simulink model "AN_Simulink_Model_v1"  (R2019b)
settings: Solver=VariableStepAuto  StartTime=0.0  StopTime=testtime  RelTol=1e-3
InitFcn:
  | AN_InitFcn_Callback
StopFcn:
  | AN_StopFcn_Callback
values from neighbouring files (symbols this model uses):
  C1initphase = C1initphase + atan(CF/(-rzero))-atan((CF-pimag(2*i-1))/(-preal(2*i-1)))-atan((CF+pimag(2*i-1))/(-preal(2*i-1)))    [AN_Get_Model_Parameters.m]
  C1slope = 0.1    [AN_Get_Model_Parameters.m]
  C2slope = 0.2    [AN_Get_Model_Parameters.m]
  CF = 2*pi*cf    [AN_Get_Model_Parameters.m]
  cordiciterationswb = 52    [AN_Get_Model_Parameters.m]
  delta_phase = -2*pi*centerfreq*tdres    [AN_Get_Model_Parameters.m]
  fs_bilinear = 2*pi*cf/tan(2*pi*cf*tdres/2)    [AN_Get_Model_Parameters.m]
  ihcasym = 3.0    (= 3)    [AN_Get_Model_Parameters.m]
  IHCLPcoeffs = [  gainihc*c2LPihc gainihc*c2LPihc 0 1 -c1LPihc 0 ... (first row only)    [AN_Get_Model_Parameters.m]
  MEcoeffs = [m14*m11 m15*m11 m16*m11 1 m12*m11 m13*m11; m24*m21 m25*m21 m26*m21 1 m22*m21 m23*m21; m34*m31 m35*m31 m36*m31 1 m32*m31 m33*m31]    [AN_Get_Model_Parameters.m]
  MEscale = 1/megainmax    (= 0.5)    [AN_Get_Model_Parameters.m]
  minR = minR    (= 0.05)    [AN_Get_Model_Parameters.m]
  norm_gainc1 = single(norm_gainc1)    [AN_Get_Model_Parameters.m]
  OHCLPcoeffs = [gainohc*c2LPohc gainohc*c2LPohc 0 1 -c1LPohc 0; gainohc*c2LPohc gainohc*c2LPohc 0 1 -c1LPohc 0]    [AN_Get_Model_Parameters.m]
  order_of_zero = half_order_pole    (= 5)    [AN_Get_Model_Parameters.m]
  pimag = zeros(11,1)    [AN_Get_Model_Parameters.m]
  preal = zeros(11,1)    [AN_Get_Model_Parameters.m]
  s0 = -dc/log(R1/(1-minR))    [AN_Get_Model_Parameters.m]
  s1 = 5.0    (= 5)    [AN_Get_Model_Parameters.m]
  shift = 1.0/(1.0+ohcasym)    (= 0.125)    [AN_Get_Model_Parameters.m]
  strength = (20.0e6)/(10^(corner/20))    (= 2000)    [AN_Get_Model_Parameters.m]
  tauwb = TauWBMax + (bmTaubm-bmTaumax)*(TauWBMax-TauWBMin)/(bmTaumax-bmTaumin)    [AN_Get_Model_Parameters.m]    (also in AN_StopFcn_Callback.m = TauWBMax+(tauc1(n+1,1)-bmTaumax)*(TauWBMax-TauWBMin)/(bmTaum)
  TauWBMax = Taumin + 0.2*(Taumax-Taumin)    [AN_Get_Model_Parameters.m]
  wborder = 3    [AN_Get_Model_Parameters.m]
  x0 = s0*log((1.0/shift-1)/(1+exp(x1/s1)))    [AN_Get_Model_Parameters.m]
  x1 = 5.0    (= 5)    [AN_Get_Model_Parameters.m]
undefined symbols (not defined in the file or in its folder): bmTaumax, bmTaumin, C2coeffs, cf, cihc, cohc, jsin, norm_gainc2, tdres, wbgain
libraries: simulink x5, dspsrcs4 x1
(part 2 of 2)

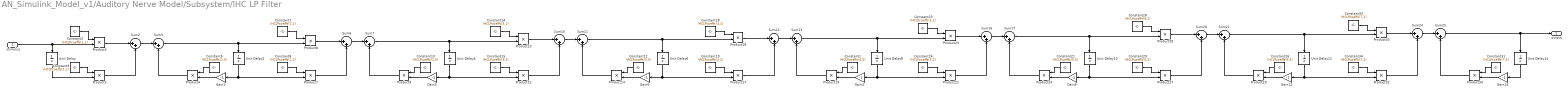
== system AN_Simulink_Model_v1/Auditory Nerve Model/Subsystem/IHC LP Filter ==
  stimulus : Inport  OutDataTypeStr=single
  Constant1 : Constant  Value=IHCLPcoeffs(4,5)  OutDataTypeStr=single  SampleTime=-1
  Constant10 : Constant  Value=IHCLPcoeffs(2,5)  OutDataTypeStr=single  SampleTime=-1
  Constant12 : Constant  Value=IHCLPcoeffs(3,5)  OutDataTypeStr=single  SampleTime=-1
  Constant14 : Constant  Value=IHCLPcoeffs(3,1)  OutDataTypeStr=single  SampleTime=-1
  Constant15 : Constant  Value=IHCLPcoeffs(3,2)  OutDataTypeStr=single  SampleTime=-1
  Constant18 : Constant  Value=IHCLPcoeffs(4,1)  OutDataTypeStr=single  SampleTime=-1
  Constant19 : Constant  Value=IHCLPcoeffs(4,2)  OutDataTypeStr=single  SampleTime=-1
  Constant2 : Constant  Value=IHCLPcoeffs(1,1)  OutDataTypeStr=single  SampleTime=-1
  Constant21 : Constant  Value=IHCLPcoeffs(5,5)  OutDataTypeStr=single  SampleTime=-1
  Constant23 : Constant  Value=IHCLPcoeffs(5,1)  OutDataTypeStr=single  SampleTime=-1
  Constant24 : Constant  Value=IHCLPcoeffs(5,2)  OutDataTypeStr=single  SampleTime=-1
  Constant26 : Constant  Value=IHCLPcoeffs(6,5)  OutDataTypeStr=single  SampleTime=-1
  Constant28 : Constant  Value=IHCLPcoeffs(6,1)  OutDataTypeStr=single  SampleTime=-1
  Constant29 : Constant  Value=IHCLPcoeffs(6,2)  OutDataTypeStr=single  SampleTime=-1
  Constant3 : Constant  Value=IHCLPcoeffs(1,2)  OutDataTypeStr=single  SampleTime=-1
  Constant31 : Constant  Value=IHCLPcoeffs(7,5)  OutDataTypeStr=single  SampleTime=-1
  Constant33 : Constant  Value=IHCLPcoeffs(7,1)  OutDataTypeStr=single  SampleTime=-1
  Constant34 : Constant  Value=IHCLPcoeffs(7,2)  OutDataTypeStr=single  SampleTime=-1
  Constant5 : Constant  Value=IHCLPcoeffs(1,5)  OutDataTypeStr=single  SampleTime=-1
  Constant7 : Constant  Value=IHCLPcoeffs(2,1)  OutDataTypeStr=single  SampleTime=-1
  Constant8 : Constant  Value=IHCLPcoeffs(2,2)  OutDataTypeStr=single  SampleTime=-1
  Gain{1,3..4,6,9,12,14} (7 alike) : Gain  Gain=-1
  Product{2..4,7..9,12..14,17..19,22..24,27..29,32..34} (21 alike) : Product
  Sum{2..3,6..7,10..13,16..17,20..21,24..25} (14 alike) : Sum  Inputs=|++
  Unit Delay{,2,4,6,8,10,12,14} (8 alike) : UnitDelay  SampleTime=-1  HasFrameUpgradeWarning=on
  output : Outport  VectorParamsAs1DForOutWhenUnconnected=off
  wires:
  Unit Delay14/1 -> Gain14/1
  Constant31/1 -> Product34/1
  Product29/1 -> Sum21/2
  Constant33/1 -> Product33/1
  Product13/1 -> Sum10/1
  Product34/1 -> Sum25/2
  Product8/1 -> Sum6/1
  Constant19/1 -> Product17/1
  Gain12/1 -> Product29/2
  Product32/1 -> Sum24/2
  Sum7/1 -> Unit Delay4/1, Product13/2
  Sum21/1 -> Unit Delay12/1, Product33/2
  Sum25/1 -> output/1, Unit Delay14/1
  Gain14/1 -> Product34/2
  Sum24/1 -> Sum25/1
  Product12/1 -> Sum10/2
  Unit Delay2/1 -> Product7/2, Gain1/1
  Unit Delay12/1 -> Product32/2, Gain12/1
  Constant26/1 -> Product29/1
  Product28/1 -> Sum20/1
  Product33/1 -> Sum24/1
  Product19/1 -> Sum13/2
  Product18/1 -> Sum12/1
  Sum16/1 -> Sum17/1
  Product27/1 -> Sum20/2
  Constant34/1 -> Product32/1
  Constant28/1 -> Product28/1
  Unit Delay10/1 -> Product27/2, Gain9/1
  Product24/1 -> Sum17/2
  Unit Delay/1 -> Product2/2
  Sum11/1 -> Unit Delay6/1, Product18/2
  Gain4/1 -> Product19/2
  Constant1/1 -> Product19/1
  stimulus/1 -> Product3/2, Unit Delay/1
  Product4/1 -> Sum3/2
  Constant24/1 -> Product22/1
  Constant21/1 -> Product24/1
  Constant29/1 -> Product27/1
  Gain9/1 -> Product24/2
  Sum20/1 -> Sum21/1
  Sum10/1 -> Sum11/1
  Gain1/1 -> Product4/2
  Unit Delay6/1 -> Product17/2, Gain6/1
  Sum12/1 -> Sum13/1
  Constant15/1 -> Product12/1
  Product14/1 -> Sum11/2
  Unit Delay8/1 -> Product22/2, Gain4/1
  Sum13/1 -> Unit Delay8/1, Product23/2
  Product17/1 -> Sum12/2
  Gain6/1 -> Product14/2
  Constant3/1 -> Product2/1
  Constant8/1 -> Product7/1
  Constant12/1 -> Product14/1
  Product3/1 -> Sum2/1
  Constant14/1 -> Product13/1
  Sum2/1 -> Sum3/1
  Sum17/1 -> Unit Delay10/1, Product28/2
  Product23/1 -> Sum16/1
  Constant10/1 -> Product9/1
  Product9/1 -> Sum7/2
  Constant2/1 -> Product3/1
  Unit Delay4/1 -> Product12/2, Gain3/1
  Product22/1 -> Sum16/2
  Constant18/1 -> Product18/1
  Constant5/1 -> Product4/1
  Constant23/1 -> Product23/1
  Constant7/1 -> Product8/1
  Sum3/1 -> Unit Delay2/1, Product8/2
  Gain3/1 -> Product9/2
  Product2/1 -> Sum2/2
  Sum6/1 -> Sum7/1
  Product7/1 -> Sum6/2

== system AN_Simulink_Model_v1/Auditory Nerve Model/Subsystem1/Calculate tauc1 ==
  note: Calculate final Time Constant which will be fed forward into C1 filter
  In1 : Inport
  Add : Sum
  Constant : Constant  Value=cohc  OutDataTypeStr=single  SampleTime=-1
  Constant1 : Constant  Value=bmTaumin  OutDataTypeStr=single  SampleTime=-1
  Constant2 : Constant  Value=bmTaumin  OutDataTypeStr=single  SampleTime=-1
  Product : Product
  Subtract : Sum  Inputs=+-
  Out1 : Outport  VectorParamsAs1DForOutWhenUnconnected=off
  wires:
  In1/1 -> Subtract/1  "tmptauc1"
  Constant/1 -> Product/1
  Constant1/1 -> Subtract/2
  Product/1 -> Add/1
  Add/1 -> Out1/1  "tauc1"
  Subtract/1 -> Product/2
  Constant2/1 -> Add/2

== system AN_Simulink_Model_v1/Auditory Nerve Model/Subsystem1/NL After OHC Function ==
  note: Ensuring Time Constant Falls within Range
  note: Nonlinear Exponential Function
  stimulus : Inport
  Abs : Abs
  Add3 : Sum
  Constant12 : Constant  Value=minR  OutDataTypeStr=single  SampleTime=-1
  Constant13 : Constant  OutDataTypeStr=single  SampleTime=-1
  Constant14 : Constant  Value=minR  OutDataTypeStr=single  SampleTime=-1
  Constant15 : Constant  Value=bmTaumax  OutDataTypeStr=single  SampleTime=-1
  Constant5 : Constant  Value=s0  OutDataTypeStr=single  SampleTime=-1
  Divide1 : Product  Inputs=*/  SaturateOnIntegerOverflow=on  RndMeth=Zero
  Exp : Math  SaturateOnIntegerOverflow=on
  Gain2 : Gain  Gain=-1
  Product3 : Product
  Product4 : Product
  Saturation : Saturate  UpperLimit=bmTaumax  LowerLimit=bmTaumin  OutDataTypeStr=single
  Subtract4 : Sum  Inputs=+-
  output : Outport  VectorParamsAs1DForOutWhenUnconnected=off
  wires:
  Saturation/1 -> output/1
  Constant12/1 -> Add3/1
  stimulus/1 -> Abs/1
  Abs/1 -> Divide1/1  "x1"
  Divide1/1 -> Gain2/1
  Constant14/1 -> Subtract4/2
  Constant15/1 -> Product4/1
  Product4/1 -> Saturation/1
  Gain2/1 -> Exp/1
  Product3/1 -> Add3/2
  Constant5/1 -> Divide1/2
  Subtract4/1 -> Product3/1
  Add3/1 -> Product4/2
  Constant13/1 -> Subtract4/1
  Exp/1 -> Product3/2

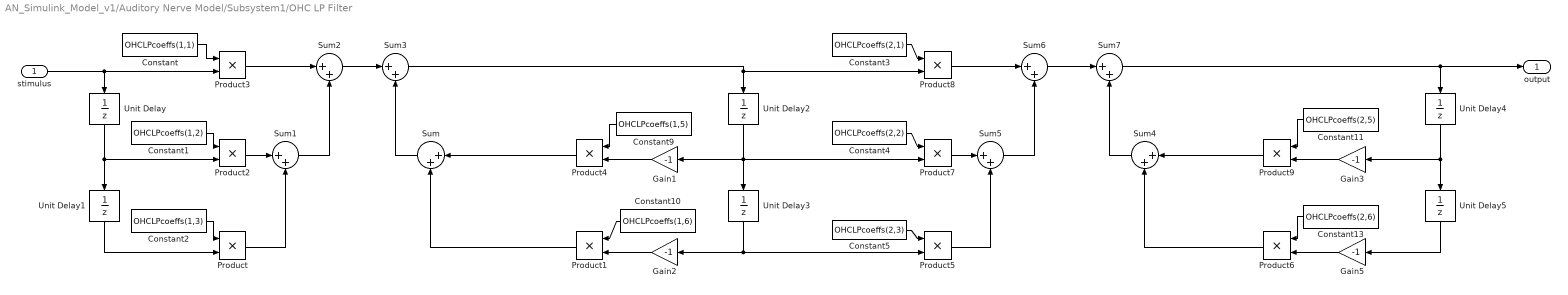
== system AN_Simulink_Model_v1/Auditory Nerve Model/Subsystem1/OHC LP Filter ==
  stimulus : Inport
  Constant : Constant  Value=OHCLPcoeffs(1,1)  OutDataTypeStr=single  SampleTime=-1
  Constant1 : Constant  Value=OHCLPcoeffs(1,2)  OutDataTypeStr=single  SampleTime=-1
  Constant10 : Constant  Value=OHCLPcoeffs(1,6)  OutDataTypeStr=single  SampleTime=-1
  Constant11 : Constant  Value=OHCLPcoeffs(2,5)  OutDataTypeStr=single  SampleTime=-1
  Constant13 : Constant  Value=OHCLPcoeffs(2,6)  OutDataTypeStr=single  SampleTime=-1
  Constant2 : Constant  Value=OHCLPcoeffs(1,3)  OutDataTypeStr=single  SampleTime=-1
  Constant3 : Constant  Value=OHCLPcoeffs(2,1)  OutDataTypeStr=single  SampleTime=-1
  Constant4 : Constant  Value=OHCLPcoeffs(2,2)  OutDataTypeStr=single  SampleTime=-1
  Constant5 : Constant  Value=OHCLPcoeffs(2,3)  OutDataTypeStr=single  SampleTime=-1
  Constant9 : Constant  Value=OHCLPcoeffs(1,5)  OutDataTypeStr=single  SampleTime=-1
  Gain{1..3,5} (4 alike) : Gain  Gain=-1
  Product{,1..9} (10 alike) : Product
  Sum{,1..7} (8 alike) : Sum  Inputs=|++
  Unit Delay{,1..5} (6 alike) : UnitDelay  SampleTime=-1  HasFrameUpgradeWarning=on
  output : Outport  VectorParamsAs1DForOutWhenUnconnected=off
  wires:
  Sum7/1 -> output/1, Unit Delay4/1
  Sum4/1 -> Sum7/2
  Constant9/1 -> Product4/1
  Unit Delay/1 -> Unit Delay1/1, Product2/2
  stimulus/1 -> Product3/2, Unit Delay/1
  Sum/1 -> Sum3/2
  Gain3/1 -> Product9/2
  Sum5/1 -> Sum6/2
  Unit Delay1/1 -> Product/2
  Product6/1 -> Sum4/2
  Product9/1 -> Sum4/1
  Product1/1 -> Sum/2
  Unit Delay5/1 -> Gain5/1
  Product4/1 -> Sum/1
  Sum2/1 -> Sum3/1
  Constant4/1 -> Product7/1
  Product/1 -> Sum1/2
  Constant11/1 -> Product9/1
  Gain2/1 -> Product1/2
  Gain5/1 -> Product6/2
  Unit Delay3/1 -> Product5/2, Gain2/1
  Gain1/1 -> Product4/2
  Constant10/1 -> Product1/1
  Constant5/1 -> Product5/1
  Product5/1 -> Sum5/2
  Product8/1 -> Sum6/1
  Constant13/1 -> Product6/1
  Product2/1 -> Sum1/1
  Constant1/1 -> Product2/1
  Constant3/1 -> Product8/1
  Sum3/1 -> Product8/2, Unit Delay2/1
  Constant/1 -> Product3/1
  Unit Delay2/1 -> Product7/2, Unit Delay3/1, Gain1/1
  Product7/1 -> Sum5/1
  Product3/1 -> Sum2/1
  Sum6/1 -> Sum7/1
  Unit Delay4/1 -> Unit Delay5/1, Gain3/1
  Sum1/1 -> Sum2/2
  Constant2/1 -> Product/1

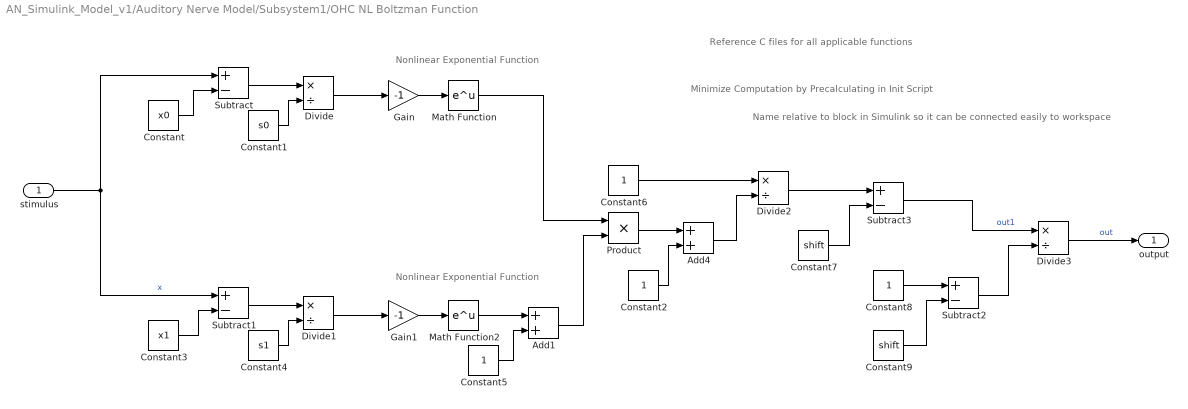
== system AN_Simulink_Model_v1/Auditory Nerve Model/Subsystem1/OHC NL Boltzman Function ==
  note: Name relative to block in Simulink so it can be connected easily to workspace
  note: Minimize Computation by Precalculating in Init Script
  note: Reference C files for all applicable functions
  note: Nonlinear Exponential Function
  note: Nonlinear Exponential Function
  stimulus : Inport
  Add1 : Sum
  Add4 : Sum
  Constant : Constant  Value=x0  OutDataTypeStr=single  SampleTime=-1
  Constant1 : Constant  Value=s0  OutDataTypeStr=single  SampleTime=-1
  Constant{2,5..6,8} (4 alike) : Constant  OutDataTypeStr=single  SampleTime=-1
  Constant3 : Constant  Value=x1  OutDataTypeStr=single  SampleTime=-1
  Constant4 : Constant  Value=s1  OutDataTypeStr=single  SampleTime=-1
  Constant7 : Constant  Value=shift  OutDataTypeStr=single  SampleTime=-1
  Constant9 : Constant  Value=shift  OutDataTypeStr=single  SampleTime=-1
  Divide{,1..3} (4 alike) : Product  Inputs=*/  SaturateOnIntegerOverflow=on  RndMeth=Zero
  Gain : Gain  Gain=-1
  Gain1 : Gain  Gain=-1
  Math Function : Math  SaturateOnIntegerOverflow=on
  Math Function2 : Math  SaturateOnIntegerOverflow=on
  Product : Product
  Subtract{,1..3} (4 alike) : Sum  Inputs=+-
  output : Outport  VectorParamsAs1DForOutWhenUnconnected=off
  wires:
  Constant/1 -> Subtract/2
  stimulus/1 -> Subtract1/1, Subtract/1  "x"
  Subtract/1 -> Divide/1
  Constant1/1 -> Divide/2
  Divide/1 -> Gain/1
  Gain/1 -> Math Function/1
  Constant3/1 -> Subtract1/2
  Subtract1/1 -> Divide1/1
  Constant4/1 -> Divide1/2
  Divide1/1 -> Gain1/1
  Gain1/1 -> Math Function2/1
  Math Function2/1 -> Add1/1
  Constant5/1 -> Add1/2
  Add1/1 -> Product/2
  Constant6/1 -> Divide2/1
  Divide2/1 -> Subtract3/1
  Constant7/1 -> Subtract3/2
  Subtract3/1 -> Divide3/1  "out1"
  Constant8/1 -> Subtract2/1
  Constant9/1 -> Subtract2/2
  Subtract2/1 -> Divide3/2
  Divide3/1 -> output/1  "out"
  Math Function/1 -> Product/1
  Product/1 -> Add4/1
  Constant2/1 -> Add4/2
  Add4/1 -> Divide2/2

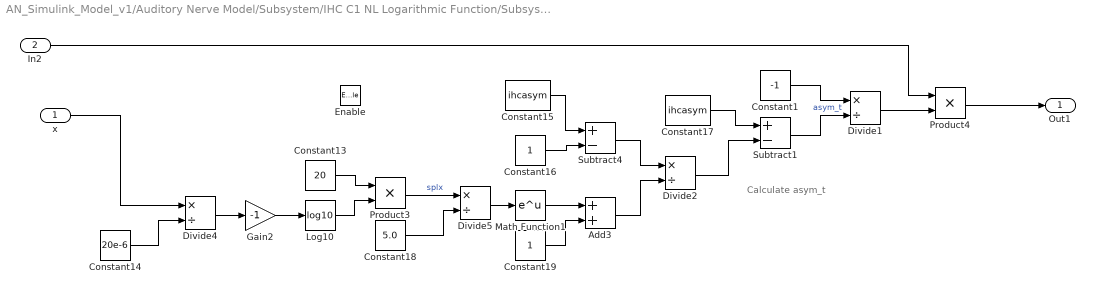
== system AN_Simulink_Model_v1/Auditory Nerve Model/Subsystem/IHC C1 NL Logarithmic Function/Subsystem1 ==
  note: Calculate asym_t
  x : Inport
  In2 : Inport  Port=2
  Enable : EnablePort
  Add3 : Sum
  Constant1 : Constant  Value=-1  OutDataTypeStr=single  SampleTime=-1
  Constant13 : Constant  Value=20  OutDataTypeStr=single  SampleTime=-1
  Constant14 : Constant  Value=20e-6  OutDataTypeStr=single  SampleTime=-1
  Constant15 : Constant  Value=ihcasym  OutDataTypeStr=single  SampleTime=-1
  Constant16 : Constant  OutDataTypeStr=single  SampleTime=-1
  Constant17 : Constant  Value=ihcasym  OutDataTypeStr=single  SampleTime=-1
  Constant18 : Constant  Value=5.0  OutDataTypeStr=single  SampleTime=-1
  Constant19 : Constant  OutDataTypeStr=single  SampleTime=-1
  Divide{1..2,4..5} (4 alike) : Product  Inputs=*/  SaturateOnIntegerOverflow=on  RndMeth=Zero
  Gain2 : Gain  Gain=-1
  Log10 : Math  Operator=log10  SaturateOnIntegerOverflow=on
  Math Function1 : Math  SaturateOnIntegerOverflow=on
  Product3 : Product
  Product4 : Product
  Subtract1 : Sum  Inputs=+-
  Subtract4 : Sum  Inputs=+-
  Out1 : Outport  OutDataTypeStr=single  InitialOutput=[0]
  wires:
  Gain2/1 -> Log10/1
  Constant13/1 -> Product3/1
  Divide5/1 -> Math Function1/1
  Math Function1/1 -> Add3/1
  Product3/1 -> Divide5/1  "splx"
  Constant15/1 -> Subtract4/1
  Log10/1 -> Product3/2
  Constant14/1 -> Divide4/2
  Constant19/1 -> Add3/2
  Divide4/1 -> Gain2/1
  Constant18/1 -> Divide5/2
  Subtract4/1 -> Divide2/1
  Constant17/1 -> Subtract1/1
  Add3/1 -> Divide2/2
  Divide2/1 -> Subtract1/2
  Subtract1/1 -> Divide1/2  "asym_t"
  Constant1/1 -> Divide1/1
  Constant16/1 -> Subtract4/2
  Divide1/1 -> Product4/2
  In2/1 -> Product4/1
  x/1 -> Divide4/1
  Product4/1 -> Out1/1

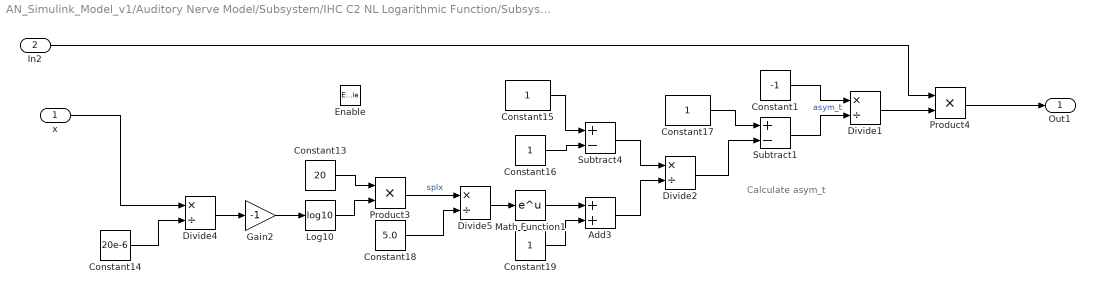
== system AN_Simulink_Model_v1/Auditory Nerve Model/Subsystem/IHC C2 NL Logarithmic Function/Subsystem1 ==
  note: Calculate asym_t
  x : Inport
  In2 : Inport  Port=2
  Enable : EnablePort
  Add3 : Sum
  Constant1 : Constant  Value=-1  OutDataTypeStr=single  SampleTime=-1
  Constant13 : Constant  Value=20  OutDataTypeStr=single  SampleTime=-1
  Constant14 : Constant  Value=20e-6  OutDataTypeStr=single  SampleTime=-1
  Constant{15..17,19} (4 alike) : Constant  OutDataTypeStr=single  SampleTime=-1
  Constant18 : Constant  Value=5.0  OutDataTypeStr=single  SampleTime=-1
  Divide{1..2,4..5} (4 alike) : Product  Inputs=*/  SaturateOnIntegerOverflow=on  RndMeth=Zero
  Gain2 : Gain  Gain=-1
  Log10 : Math  Operator=log10  SaturateOnIntegerOverflow=on
  Math Function1 : Math  SaturateOnIntegerOverflow=on
  Product3 : Product
  Product4 : Product
  Subtract1 : Sum  Inputs=+-
  Subtract4 : Sum  Inputs=+-
  Out1 : Outport  OutDataTypeStr=single  InitialOutput=[0]
  wires:
  Gain2/1 -> Log10/1
  Constant13/1 -> Product3/1
  Divide5/1 -> Math Function1/1
  Math Function1/1 -> Add3/1
  Product3/1 -> Divide5/1  "splx"
  Constant15/1 -> Subtract4/1
  Log10/1 -> Product3/2
  Constant14/1 -> Divide4/2
  Constant19/1 -> Add3/2
  Divide4/1 -> Gain2/1
  Constant18/1 -> Divide5/2
  Subtract4/1 -> Divide2/1
  Constant17/1 -> Subtract1/1
  Add3/1 -> Divide2/2
  Divide2/1 -> Subtract1/2
  Subtract1/1 -> Divide1/2  "asym_t"
  Constant1/1 -> Divide1/1
  Constant16/1 -> Subtract4/2
  Divide1/1 -> Product4/2
  In2/1 -> Product4/1
  x/1 -> Divide4/1
  Product4/1 -> Out1/1

== matlab function AN_Simulink_Model_v1/Auditory Nerve Model/CP Wideband Gammatone Filter/MATLAB Function1 ==
  data: phase input; wbphase output; delta_phase input
% Matthew Blunt
% Speech % Hearing Internship
% Check Gammatone Cosine Argument
% 6/6/2019

% ---------------------------------------------------------------------- %
% NOTES: 
% ---------------------------------------------------------------------- %

% The following script is designed to work within the CP Wideband Gammatone
% Filter Simulink model in order to ensure that the argument of the
% trigonometric representation of a complex exponential remains within
% [-2pi,2pi). The function will simply take in the wb phase variable and
% output the same value in radians that falls within the range of arguments
% for the Simulink trigonometric block.

% *** NOTE: Edited by Matthew Blunt 03/05/2020
% *** Now evaluates bounds in the feedback loop to ensure stability for
% FPGA implementation

% ---------------------------------------------------------------------- %
% CODE: 
% ---------------------------------------------------------------------- %

% *** Edited by Matthew Blunt 03/05/2020
% *** Only accounts for negative values of delta_phase
function wbphase = WbGammaToneCosineArgCheck(phase,delta_phase)
    if phase <= (-2*pi - delta_phase)
        phase = phase+2*pi;
    end
    wbphase = phase;
end
